simulink model "LM"  (R2013a)
settings: Solver=ode45  StartTime=0.0  StopTime=30.0  RelTol=1e-3
libraries: simulink x1
settings Model: Creator=Labo  LastModifiedBy=Labo

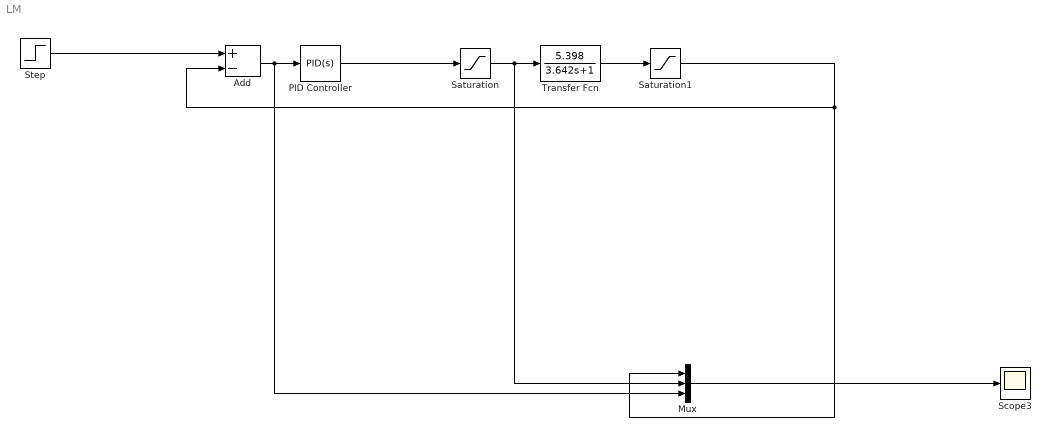
== system LM ==
  Add : Sum  Inputs=+-
  Mux : Mux  Inputs=3
  PID Controller : simulink/Continuous/PID Controller  Controller=PID  TimeDomain=Continuous-time  SampleTime=1  IntegratorMethod=Forward Euler  FilterMethod=Forward Euler  Form=Parallel  P=1.44  I=1.44/3.642  D=0  N=100  InitialConditionSource=internal  InitialConditionForIntegrator=0  InitialConditionForFilter=0  ExternalReset=none  LimitOutput=off  UpperSaturationLimit=inf  LowerSaturationLimit=-inf  LinearizeAsGain=on  AntiWindupMode=none  Kb=1  TrackingMode=off  Kt=1  PParamMin=[]  PParamMax=[]  IParamMin=[]  IParamMax=[]  DParamMin=[]  DParamMax=[]  NParamMin=[]  NParamMax=[]  KbParamMin=[]  KbParamMax=[]  KtParamMin=[]  KtParamMax=[]  POutMin=[]  POutMax=[]  IOutMin=[]  IOutMax=[]  DOutMin=[]  DOutMax=[]  NOutMin=[]  NOutMax=[]  KbOutMin=[]  KbOutMax=[]  KtOutMin=[]  KtOutMax=[]  IntegratorOutMin=[]  IntegratorOutMax=[]  FilterOutMin=[]  FilterOutMax=[]  SumOutMin=[]  SumOutMax=[]  SumI1OutMin=[]  SumI1OutMax=[]  SumI2OutMin=[]  SumI2OutMax=[]  SumI3OutMin=[]  SumI3OutMax=[]  SumDOutMin=[]  SumDOutMax=[]  SaturationOutMin=[]  SaturationOutMax=[]  IntegratorContinuousStateAttributes=''  IntegratorStateMustResolveToSignalObject=off  IntegratorRTWStateStorageClass=Auto  FilterContinuousStateAttributes=''  FilterStateMustResolveToSignalObject=off  FilterRTWStateStorageClass=Auto
  Saturation : Saturate  UpperLimit=7.3  LowerLimit=-17.3
  Saturation1 : Saturate  UpperLimit=10-8.623  LowerLimit=-10-8.623
  Scope3 : Scope
  Step : Step  After=0.15  SampleTime=0
  Transfer Fcn : TransferFcn  Numerator=[5.398]  Denominator=[3.642 1]  ContinuousStateAttributes='v'
  wires:
  Add/1 -> Mux/3, PID Controller/1
  Transfer Fcn/1 -> Saturation1/1
  Saturation1/1 -> Mux/1, Add/2
  Saturation/1 -> Mux/2, Transfer Fcn/1
  Mux/1 -> Scope3/1
  Step/1 -> Add/1
  PID Controller/1 -> Saturation/1
